simulink model "vocoder_v2"  (R2020a)
settings: Solver=FixedStepDiscrete  StartTime=0.0  StopTime=inf  RelTol=1e-3
libraries: dspvision x2, audiosources x1, dspsnks4 x1
settings Model: Creator=unity  LastModifiedBy=unity
settings SolverCC: AutoInsertRateTranBlk=on
settings DataIOCC: LimitDataPoints=on  SaveOutput=off  SignalLogging=off  SaveTime=off
settings OptimizationCC: LifeSpan=inf
settings DebuggingCC: AlgebraicLoopMsg=error  SingleTaskRateTransMsg=error  AllowSymbolicDim=off  SFUnexpectedBacktrackingDiag=warning  SFNoUnconditionalDefaultTransitionDiag=warning  SFExecutionAtInitializationDiag=none  ArithmeticOperatorsInVariantConditions=warning
settings SFSimCC: SimUseLocalCustomCode=off  CustomCodeUndefinedFunction=UseInterfaceOnly
settings RTWCC: RTWUseLocalCustomCode=off
settings CodeAppCC: StateflowObjectComments=on
settings GRTTargetCC: TargetLangStandard=C89/C90 (ANSI)
settings ConfigComp: CovMetricSettings=dw  CovHtmlReporting=on  CovSaveCumulativeToWorkspaceVar=on  CovSaveSingleToWorkspaceVar=on  CovExternalEMLEnable=off  CovSFcnEnable=off

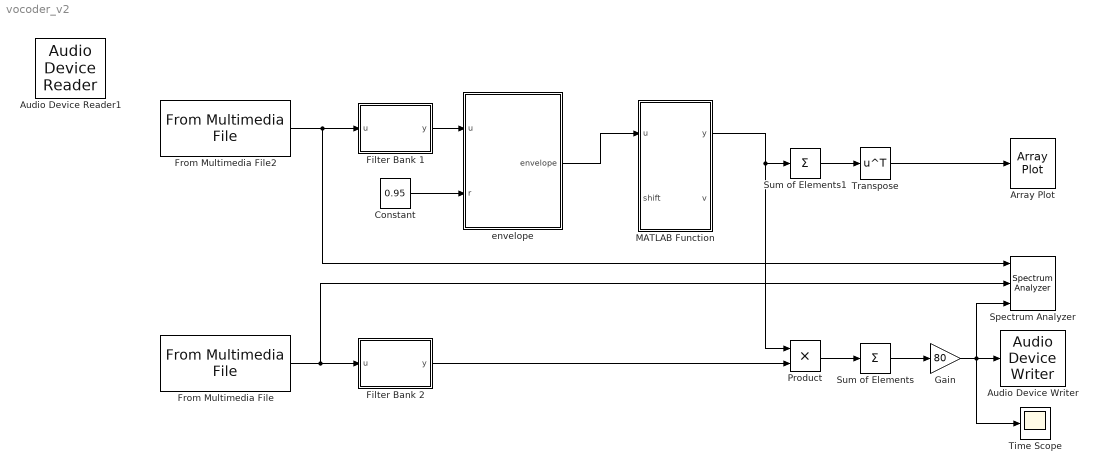
== system vocoder_v2 ==
  Array Plot : ArrayPlot
  Audio Device Reader1 : audiosources/Audio Device Reader  Driver=DirectSound  Device=Default  SampleRate=44100  NumChannels=1  SamplesPerFrame=1024  BitDepth=16-bit integer  NumBuffers=10  DefaultInputChannelMapping=on  InputChannelMapping=1:2  OutputNumOverrunSamples=off  OutputDataType=double  DriverIdx=1  DeviceWarnFlag=''
      settings: SourceProductBaseCode=AU
  Audio Device Writer : dspsnks4/Audio Device Writer  Driver=DirectSound  Device=Default  InheritSampleRate=on  SampleRate=44100  BitDepth=16-bit integer  BufferSize=4096  NumBuffers=10  DefaultOutputChannelMapping=on  OutputChannelMapping=1:2  OutputNumUnderrunSamples=off  DriverIdx=1  DeviceWarnFlag=''
  Constant : Constant  Value=0.95
  Filter Bank 1 : MATLAB Function  TreatAsAtomicUnit=on
  Filter Bank 2 : MATLAB Function  TreatAsAtomicUnit=on
  From Multimedia File : dspvision/From Multimedia File  inputFilename=D:\github\matlab_audio\vocoder\audio\synth.wav  readRange=[1 Inf]  loop=on  numPlays=inf  outputStreams=オーディオのみ  videoDataType=single  audioDataType=double  inheritSampleTime=on  userDefinedSampleTime=1/30  noAudioOutput=off  isIntensityVideo=off  fourcc=RGB  colorVideoFormat=Separate color signals  outputEOF=off  dataOrg=Column-major  audioFrameSize=1024  computeAudioFrameSize=off  outSamplingMode=Sample based
  From Multimedia File2 : dspvision/From Multimedia File  inputFilename=D:\github\matlab_audio\vocoder\audio\voice.wav  readRange=[1 Inf]  loop=on  numPlays=inf  outputStreams=オーディオのみ  videoDataType=single  audioDataType=double  inheritSampleTime=on  userDefinedSampleTime=1/30  noAudioOutput=off  isIntensityVideo=off  fourcc=RGB  colorVideoFormat=Separate color signals  outputEOF=off  dataOrg=Column-major  audioFrameSize=1024  computeAudioFrameSize=off  outSamplingMode=Sample based
  Gain : Gain  Gain=80
  MATLAB Function : MATLAB Function  TreatAsAtomicUnit=on
  Product : Product
  Spectrum Analyzer : SpectrumAnalyzer  NumInputPorts=3
  Sum of Elements : Sum  Inputs=+  CollapseMode=Specified dimension  CollapseDim=2
  Sum of Elements1 : Sum  Inputs=+  CollapseMode=Specified dimension
  Time Scope : Scope
  Transpose : Math  Operator=transpose  SaturateOnIntegerOverflow=on
  envelope : MATLAB Function  TreatAsAtomicUnit=on
  wires:
  Filter Bank 1/1(y) -> envelope/1(u)
  Constant/1 -> envelope/2(r)
  Filter Bank 2/1(y) -> Product/2
  envelope/1(envelope) -> MATLAB Function/1(u)
  Product/1 -> Sum of Elements/1
  Sum of Elements/1 -> Gain/1
  Sum of Elements1/1 -> Transpose/1
  Transpose/1 -> Array Plot/1
  From Multimedia File2/1 -> Filter Bank 1/1(u), Spectrum Analyzer/1
  From Multimedia File/1 -> Filter Bank 2/1(u), Spectrum Analyzer/2
  Gain/1 -> Spectrum Analyzer/3, Time Scope/1, Audio Device Writer/1
  MATLAB Function/1(y) -> Product/1, Sum of Elements1/1

== matlab function vocoder_v2/Filter Bank 2 ==
  data: u input; y output
function y = fcn(u)
    Fs = 44.1*10^3;
    N = 4;
    persistent ofb
    if isempty(ofb)
        ofb = octaveFilterBank('1/12 octave',Fs,'FilterOrder',N);
    end
    y = ofb(u);

== matlab function vocoder_v2/Filter Bank 1 ==
  data: u input; y output
function y = fcn(u)
    Fs = 44.1*10^3;
    N = 4;
    persistent ofb
    if isempty(ofb)
        ofb = octaveFilterBank('1/12 octave',Fs,'FilterOrder',N);
    end
    y = ofb(u);

== matlab function vocoder_v2/envelope ==
  data: u input; envelope output; r input
function envelope = fcn(u,r)
    [n_bands,frame_size]=size(u);
    u = abs(u);
    envelope = zeros(n_bands,frame_size);
    
    persistent level
    if isempty(level)
        level = zeros(n_bands);
    end
    
    for band = 1:n_bands
        for i = 1:frame_size
            if level(band) < u(band,i)
                level(band) = u(band,i);
            else
                level(band) = level(band)*r;
            end
            envelope(band,i) = level(band);
        end
    end
end

== matlab function vocoder_v2/MATLAB Function ==
  data: u input; y output; shift input; v output
function [y,v] = fcn(u,shift)
    [n_bands,frame_size]=size(u);
    v = cat(2,cat(2,zeros(n_bands,frame_size),u),zeros(n_bands,frame_size));
    
    shift = shift*6;
    int_index = frame_size;
y = u;
